simulink model "p_control"  (R2019b)
settings: Solver=VariableStepAuto  StartTime=0.0  StopTime=10.0  RelTol=1e-3
settings Model: Creator=bsb  LastModifiedBy=bsb

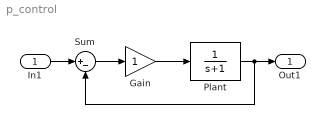
== system p_control ==
  In1 : Inport
      mask Display: disp('R(s)')
  Gain : Gain
      mask Display: disp('K_p','interpreter','tex')
  Plant : TransferFcn  Numerator=1  Denominator=[1 1]  ContinuousStateAttributes='theta'
      mask Display: disp('G(s)')
  Sum : Sum  Inputs=|+-
  Out1 : Outport
      mask Display: disp('C(s)')
  wires:
  Plant/1 -> Sum/2, Out1/1
  Gain/1 -> Plant/1
  In1/1 -> Sum/1
  Sum/1 -> Gain/1
